simulink model "bitcrusher_ref"  (R2020b)
settings: Solver=FixedStepDiscrete  StartTime=0.0  StopTime=stopTime  FixedStep=1.0416666666666666e-05  RelTol=1e-3
libraries: simulink x2
settings Model: Creator=Ross  LastModifiedBy=wickh
settings DataIOCC: SaveOutput=off  SaveTime=off  ReturnWorkspaceOutputs=off
settings OptimizationCC: BlockReduction=off  ConditionallyExecuteInputs=off  DefaultParameterBehavior=Inlined
settings DebuggingCC: ReadBeforeWriteMsg=DisableAll  WriteAfterWriteMsg=DisableAll  WriteAfterReadMsg=DisableAll  AlgebraicLoopMsg=error  MultiTaskDSMMsg=none  SingleTaskRateTransMsg=error  PregeneratedLibrarySubsystemCodeDiagnostic=none  ArithmeticOperatorsInVariantConditions=warning
settings HardwareCC: ProdBitPerPointer=32  ProdBitPerSizeT=32  ProdBitPerPtrDiffT=32  ProdLargestAtomicFloat=None  ProdIntDivRoundTo=Undefined  ProdEndianess=Unspecified  ProdWordSize=32  ProdHWDeviceType=ASIC/FPGA->ASIC/FPGA  TargetBitPerPointer=64  TargetBitPerSizeT=64  TargetBitPerPtrDiffT=64  TargetLongLongMode=on  TargetIntDivRoundTo=Zero  TargetEndianess=LittleEndian  TargetWordSize=64  TargetHWDeviceType=Custom Processor->MATLAB Host Computer  ProdEqTarget=off
settings ModelReferenceCC: UpdateModelReferenceTargets=IfOutOfDate
settings SFSimCC: SFSimEcho=off  SimUseLocalCustomCode=off  CustomCodeUndefinedFunction=UseInterfaceOnly
settings RTWCC: RTWUseLocalCustomCode=off

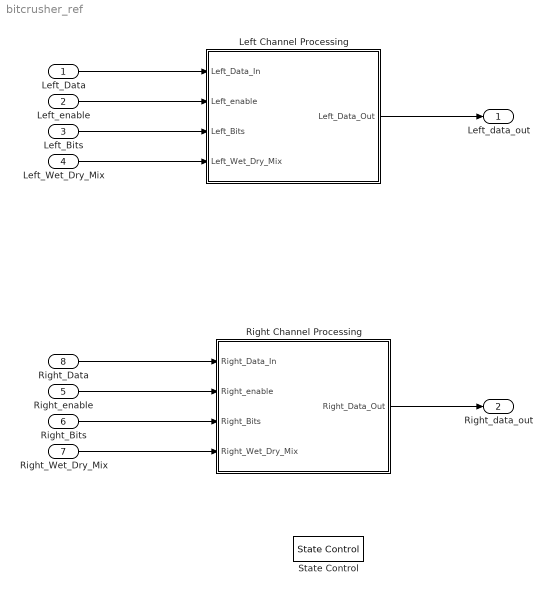
== system bitcrusher_ref ==
  Left_Data : Inport  OutDataTypeStr=fixdt(1,24,23)  PortDimensions=1
  Left_enable : Inport  Port=2  OutDataTypeStr=boolean  PortDimensions=1  SampleTime=[1.0416666666666666e-05,0]
  Left_Bits : Inport  Port=3  OutDataTypeStr=fixdt(0,5,0)  PortDimensions=1  SampleTime=[1.0416666666666666e-05,0]
  Left_Wet_Dry_Mix : Inport  Port=4  OutDataTypeStr=fixdt(0,8,7)  PortDimensions=1  SampleTime=[1.0416666666666666e-05,0]
  Right_enable : Inport  Port=5  OutDataTypeStr=boolean  PortDimensions=1  SampleTime=[1.0416666666666666e-05,0]
  Right_Bits : Inport  Port=6  OutDataTypeStr=fixdt(0,5,0)  PortDimensions=1  SampleTime=[1.0416666666666666e-05,0]
  Right_Wet_Dry_Mix : Inport  Port=7  OutDataTypeStr=fixdt(0,8,7)  PortDimensions=1  SampleTime=[1.0416666666666666e-05,0]
  Right_Data : Inport  Port=8  OutDataTypeStr=fixdt(1,24,23)  PortDimensions=1
  Left Channel Processing : Subsystem  TreatAsAtomicUnit=on
  Right Channel Processing : Subsystem  TreatAsAtomicUnit=on
  State Control : StateControl  StateControl=Synchronous
  Left_data_out : Outport  OutDataTypeStr=fixdt(1,24,23)  PortDimensions=1  InitialOutput=0  VectorParamsAs1DForOutWhenUnconnected=off
  Right_data_out : Outport  Port=2  OutDataTypeStr=fixdt(1,24,23)  PortDimensions=1  InitialOutput=0  VectorParamsAs1DForOutWhenUnconnected=off
  wires:
  Right Channel Processing/1("Right_Data_Out ") -> Right_data_out/1
  Left Channel Processing/1("Left_Data_Out ") -> Left_data_out/1
  Left_Bits/1 -> Left Channel Processing/3(Left_Bits)
  Right_Bits/1 -> Right Channel Processing/3(Right_Bits)
  Left_enable/1 -> Left Channel Processing/2(Left_enable)
  Right_enable/1 -> Right Channel Processing/2(Right_enable)
  Left_Wet_Dry_Mix/1 -> Left Channel Processing/4(Left_Wet_Dry_Mix)
  Right_Wet_Dry_Mix/1 -> Right Channel Processing/4(Right_Wet_Dry_Mix)
  Left_Data/1 -> Left Channel Processing/1(Left_Data_In)
  Right_Data/1 -> Right Channel Processing/1(Right_Data_In)

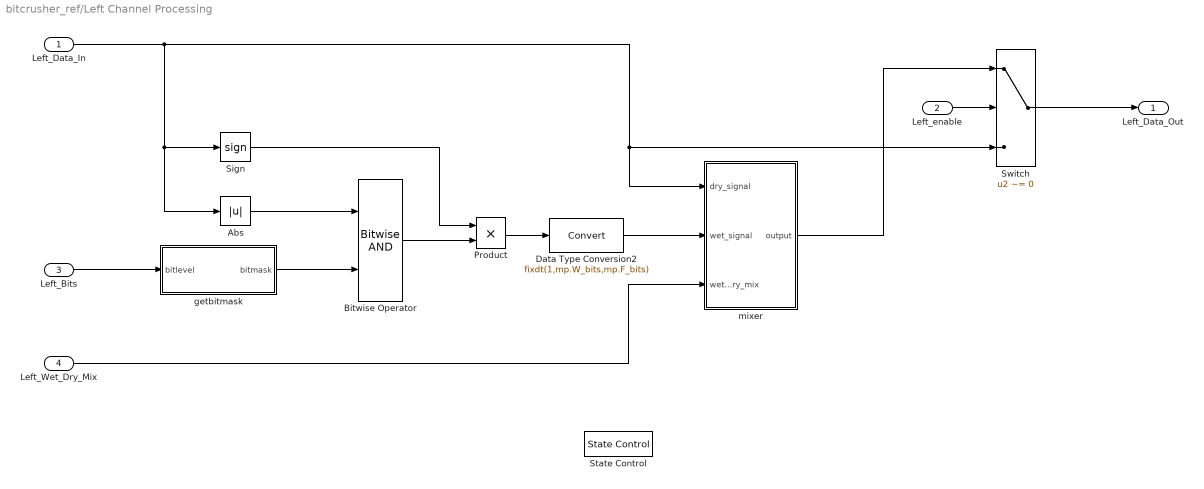
== system bitcrusher_ref/Left Channel Processing ==
  Left_Data_In : Inport
  Left_enable : Inport  Port=2
  Left_Bits : Inport  Port=3
  Left_Wet_Dry_Mix : Inport  Port=4
  Abs : Abs  OutDataTypeStr=fixdt(0,32,28)
  Bitwise Operator : simulink/Logic and Bit Operations/Bitwise Operator  logicop=AND  UseBitMask=off  NumInputPorts=2  BitMask=bin2dec('11011001')  BitMaskRealWorld=Stored Integer
  Data Type Conversion2 : DataTypeConversion  OutDataTypeStr=fixdt(1,mp.W_bits,mp.F_bits)
  Product : Product
  Sign : Signum
  State Control : StateControl  StateControl=Synchronous
  Switch : Switch  Criteria=u2 ~= 0
  getbitmask : MATLAB Function  TreatAsAtomicUnit=on
  mixer : Subsystem
  "Left_Data_Out " : Outport  InitialOutput=0  VectorParamsAs1DForOutWhenUnconnected=off
  wires:
  mixer/1(output) -> Switch/1
  Left_enable/1 -> Switch/2
  Left_Wet_Dry_Mix/1 -> mixer/3(wet_dry_mix)
  Data Type Conversion2/1 -> mixer/2(wet_signal)
  Switch/1 -> "Left_Data_Out "/1
  Sign/1 -> Product/1
  Bitwise Operator/1 -> Product/2
  Product/1 -> Data Type Conversion2/1
  Abs/1 -> Bitwise Operator/1
  Left_Data_In/1 -> Switch/3, mixer/1(dry_signal), Sign/1, Abs/1
  getbitmask/1(bitmask) -> Bitwise Operator/2
  Left_Bits/1 -> getbitmask/1(bitlevel)

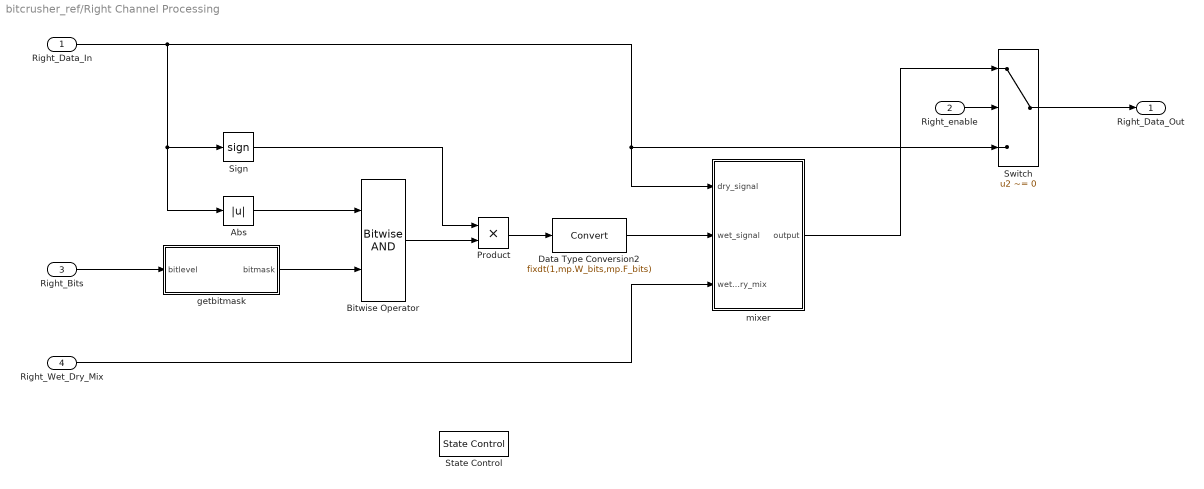
== system bitcrusher_ref/Right Channel Processing ==
  Right_Data_In : Inport
  Right_enable : Inport  Port=2
  Right_Bits : Inport  Port=3
  Right_Wet_Dry_Mix : Inport  Port=4
  Abs : Abs  OutDataTypeStr=fixdt(0,32,28)
  Bitwise Operator : simulink/Logic and Bit Operations/Bitwise Operator  logicop=AND  UseBitMask=off  NumInputPorts=2  BitMask=bin2dec('11011001')  BitMaskRealWorld=Stored Integer
  Data Type Conversion2 : DataTypeConversion  OutDataTypeStr=fixdt(1,mp.W_bits,mp.F_bits)
  Product : Product
  Sign : Signum
  State Control : StateControl  StateControl=Synchronous
  Switch : Switch  Criteria=u2 ~= 0
  getbitmask : MATLAB Function  TreatAsAtomicUnit=on
  mixer : Subsystem
  "Right_Data_Out " : Outport  InitialOutput=0  VectorParamsAs1DForOutWhenUnconnected=off
  wires:
  Right_enable/1 -> Switch/2
  mixer/1(output) -> Switch/1
  Right_Wet_Dry_Mix/1 -> mixer/3(wet_dry_mix)
  Data Type Conversion2/1 -> mixer/2(wet_signal)
  Switch/1 -> "Right_Data_Out "/1
  Sign/1 -> Product/1
  Bitwise Operator/1 -> Product/2
  Product/1 -> Data Type Conversion2/1
  Abs/1 -> Bitwise Operator/1
  Right_Data_In/1 -> mixer/1(dry_signal), Switch/3, Sign/1, Abs/1
  getbitmask/1(bitmask) -> Bitwise Operator/2
  Right_Bits/1 -> getbitmask/1(bitlevel)

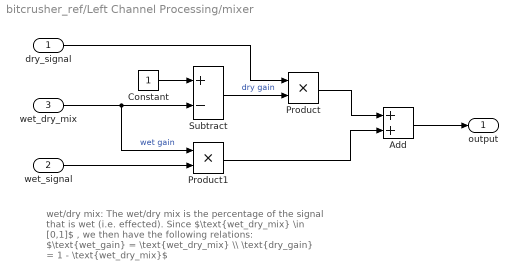
== system bitcrusher_ref/Left Channel Processing/mixer ==
  note: wet/dry mix:
      | The wet/dry mix is the percentage of the signal that is wet (i.e. effected).
      |
      | Since $\text{wet_dry_mix} \in [0,1]$ , we then have the following relations:
      | $\text{wet_gain} = \text{wet_dry_mix} \\ \text{dry_gain} = 1 - \text{wet_dry_mix}$
  dry_signal : Inport
  wet_signal : Inport  Port=2
  wet_dry_mix : Inport  Port=3
  Add : Sum  OutDataTypeStr=fixdt(1,mp.W_bits,mp.F_bits)
  Constant : Constant  OutDataTypeStr=Inherit: Inherit via back propagation  SampleTime=-1
  Product : Product  OutDataTypeStr=Inherit: Keep MSB
  Product1 : Product  OutDataTypeStr=Inherit: Keep MSB
  Subtract : Sum  Inputs=+-  InputSameDT=on  OutDataTypeStr=Inherit: Same as first input
  output : Outport  VectorParamsAs1DForOutWhenUnconnected=off
  wires:
  Subtract/1 -> Product/2  "dry gain"
  dry_signal/1 -> Product/1
  wet_signal/1 -> Product1/2
  Product1/1 -> Add/2
  Product/1 -> Add/1
  wet_dry_mix/1 -> Subtract/2, Product1/1  "wet gain"
  Constant/1 -> Subtract/1
  Add/1 -> output/1

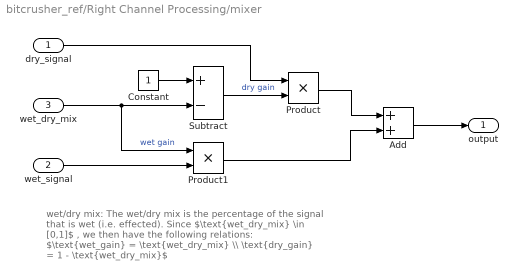
== system bitcrusher_ref/Right Channel Processing/mixer ==
  note: wet/dry mix:
      | The wet/dry mix is the percentage of the signal that is wet (i.e. effected).
      |
      | Since $\text{wet_dry_mix} \in [0,1]$ , we then have the following relations:
      | $\text{wet_gain} = \text{wet_dry_mix} \\ \text{dry_gain} = 1 - \text{wet_dry_mix}$
  dry_signal : Inport
  wet_signal : Inport  Port=2
  wet_dry_mix : Inport  Port=3
  Add : Sum  OutDataTypeStr=fixdt(1,mp.W_bits,mp.F_bits)
  Constant : Constant  OutDataTypeStr=Inherit: Inherit via back propagation  SampleTime=-1
  Product : Product  OutDataTypeStr=Inherit: Keep MSB
  Product1 : Product  OutDataTypeStr=Inherit: Keep MSB
  Subtract : Sum  Inputs=+-  InputSameDT=on  OutDataTypeStr=Inherit: Same as first input
  output : Outport  VectorParamsAs1DForOutWhenUnconnected=off
  wires:
  wet_signal/1 -> Product1/2
  Add/1 -> output/1
  Constant/1 -> Subtract/1
  wet_dry_mix/1 -> Subtract/2, Product1/1  "wet gain"
  Subtract/1 -> Product/2  "dry gain"
  dry_signal/1 -> Product/1
  Product/1 -> Add/1
  Product1/1 -> Add/2

== matlab function bitcrusher_ref/Left Channel Processing/getbitmask ==
  data: bitlevel input; bitmask output
function bitmask = getbitmask(bitlevel)
bitmask=fi(0,0,32,28);
switch(bitlevel)
    case 0
        bitmask = fi(0.0000000000000000000000000000,0,32,28);
    case 1
        bitmask = fi(8.0000000000000000000000000000,0,32,28);
    case 2
        bitmask = fi(12.0000000000000000000000000000,0,32,28);
    case 3
        bitmask = fi(14.0000000000000000000000000000,0,32,28);
    case 4
        bitmask = fi(15.0000000000000000000000000000,0,32,28);
    case 5
        bitmask = fi(15.5000000000000000000000000000,0,32,28);
    case 6
        bitmask = fi(15.7500000000000000000000000000,0,32,28);
    case 7
        bitmask = fi(15.8750000000000000000000000000,0,32,28);
    case 8
        bitmask = fi(15.9375000000000000000000000000,0,32,28);
    case 9
        bitmask = fi(15.9687500000000000000000000000,0,32,28);
    case 10
        bitmask = fi(15.9843750000000000000000000000,0,32,28);
    case 11
        bitmask = fi(15.9921875000000000000000000000,0,32,28);
    case 12
        bitmask = fi(15.9960937500000000000000000000,0,32,28);
    case 13
        bitmask = fi(15.9980468750000000000000000000,0,32,28);
    case 14
        bitmask = fi(15.9990234375000000000000000000,0,32,28);
    case 15
        bitmask = fi(15.9995117187500000000000000000,0,32,28);
    case 16
        bitmask = fi(15.9997558593750000000000000000,0,32,28);
    case 17
        bitmask = fi(15.9998779296875000000000000000,0,32,28);
    case 18
        bitmask = fi(15.9999389648437500000000000000,0,32,28);
    case 19
        bitmask = fi(15.9999694824218750000000000000,0,32,28);
    case 20
        bitmask = fi(15.9999847412109375000000000000,0,32,28);
    case 21
        bitmask = fi(15.9999923706054687500000000000,0,32,28);
    case 22
        bitmask = fi(15.9999961853027343750000000000,0,32,28);
    case 23
        bitmask = fi(15.9999980926513671875000000000,0,32,28);
    case 24
        bitmask = fi(15.9999990463256835937500000000,0,32,28);
    case 25
        bitmask = fi(15.9999995231628417968750000000,0,32,28);
    case 26
        bitmask = fi(15.9999997615814208984375000000,0,32,28);
    case 27
        bitmask = fi(15.9999998807907104492187500000,0,32,28);
    case 28
        bitmask = fi(15.9999999403953552246093750000,0,32,28);
    case 29
        bitmask = fi(15.9999999701976776123046875000,0,32,28);
    case 30
        bitmask = fi(15.9999999850988388061523437500,0,32,28);
    case 31
        bitmask = fi(15.9999999925494194030761718750,0,32,28);
    case 32
        bitmask = fi(15.9999999962747097015380859375,0,32,28);
end

== matlab function bitcrusher_ref/Right Channel Processing/getbitmask ==
  data: bitlevel input; bitmask output
function bitmask = getbitmask(bitlevel)
bitmask=fi(0,0,32,28);
switch(bitlevel)
    case 0
        bitmask = fi(0.0000000000000000000000000000,0,32,28);
    case 1
        bitmask = fi(8.0000000000000000000000000000,0,32,28);
    case 2
        bitmask = fi(12.0000000000000000000000000000,0,32,28);
    case 3
        bitmask = fi(14.0000000000000000000000000000,0,32,28);
    case 4
        bitmask = fi(15.0000000000000000000000000000,0,32,28);
    case 5
        bitmask = fi(15.5000000000000000000000000000,0,32,28);
    case 6
        bitmask = fi(15.7500000000000000000000000000,0,32,28);
    case 7
        bitmask = fi(15.8750000000000000000000000000,0,32,28);
    case 8
        bitmask = fi(15.9375000000000000000000000000,0,32,28);
    case 9
        bitmask = fi(15.9687500000000000000000000000,0,32,28);
    case 10
        bitmask = fi(15.9843750000000000000000000000,0,32,28);
    case 11
        bitmask = fi(15.9921875000000000000000000000,0,32,28);
    case 12
        bitmask = fi(15.9960937500000000000000000000,0,32,28);
    case 13
        bitmask = fi(15.9980468750000000000000000000,0,32,28);
    case 14
        bitmask = fi(15.9990234375000000000000000000,0,32,28);
    case 15
        bitmask = fi(15.9995117187500000000000000000,0,32,28);
    case 16
        bitmask = fi(15.9997558593750000000000000000,0,32,28);
    case 17
        bitmask = fi(15.9998779296875000000000000000,0,32,28);
    case 18
        bitmask = fi(15.9999389648437500000000000000,0,32,28);
    case 19
        bitmask = fi(15.9999694824218750000000000000,0,32,28);
    case 20
        bitmask = fi(15.9999847412109375000000000000,0,32,28);
    case 21
        bitmask = fi(15.9999923706054687500000000000,0,32,28);
    case 22
        bitmask = fi(15.9999961853027343750000000000,0,32,28);
    case 23
        bitmask = fi(15.9999980926513671875000000000,0,32,28);
    case 24
        bitmask = fi(15.9999990463256835937500000000,0,32,28);
    case 25
        bitmask = fi(15.9999995231628417968750000000,0,32,28);
    case 26
        bitmask = fi(15.9999997615814208984375000000,0,32,28);
    case 27
        bitmask = fi(15.9999998807907104492187500000,0,32,28);
    case 28
        bitmask = fi(15.9999999403953552246093750000,0,32,28);
    case 29
        bitmask = fi(15.9999999701976776123046875000,0,32,28);
    case 30
        bitmask = fi(15.9999999850988388061523437500,0,32,28);
    case 31
        bitmask = fi(15.9999999925494194030761718750,0,32,28);
    case 32
        bitmask = fi(15.9999999962747097015380859375,0,32,28);
end
